simulink model "my_safety"  (R2023b)
settings: Solver=FixedStepAuto  StartTime=0.0  StopTime=inf  RelTol=1e-3
undefined symbols (not defined in the file): Alt, Button, Lat, Lon, recfin, Xa, Ya, Yg, Za
libraries: simulink x12, androiduilib x8, androidsensorlib x3, androidaudiovideolib x2, androidcommunicationlib x1
settings Model: Creator=salon  LastModifiedBy=salon
settings OptimizationCC: EnhancedBackFolding=on  PassReuseOutputArgsAs=Individual arguments  ZeroExternalMemoryAtStartup=off  ZeroInternalMemoryAtStartup=off  MaxStackSize=64  OptimizeBlockOrder=speed  DifferentSizesBufferReuse=on  OptimizationCustomize=off  EfficientTunableParamExpr=on
settings DebuggingCC: ParameterTunabilityLossMsg=error
settings HardwareCC: ProdBitPerPointer=32  ProdBitPerSizeT=32  ProdBitPerPtrDiffT=32  ProdLargestAtomicInteger=Long  ProdLargestAtomicFloat=Double  ProdWordSize=32  ProdHWDeviceType=ARM Compatible->ARM Cortex  UseEmbeddedCoderFeatures=off  UseSimulinkCoderFeatures=off
settings SFSimCC: MATLABDynamicMemAlloc=off
settings RTWCC: Description=Embedded Coder  SystemTargetFile=ert.tlc  HardwareBoard=Android Device  TLCOptions="-aInlineSetEventsForThisBaseRateFcn=TLC_FALSE -aSuppressMultiTaskScheduler=TLC_FALSE  -aRateBasedStepFcn=0"  TemplateMakefile=ert_default_tmf  RTWVerbose=off  Toolchain=Android SDK/NDK Tools
settings CodeAppCC: ForceParamTrailComments=on  IgnoreCustomStorageClasses=off  OperatorAnnotations=on  SimulinkDataObjDesc=on  SFDataObjDesc=on  InsertBlockDesc=on
settings ERTTargetCC: SupportNonInlinedSFcns=on

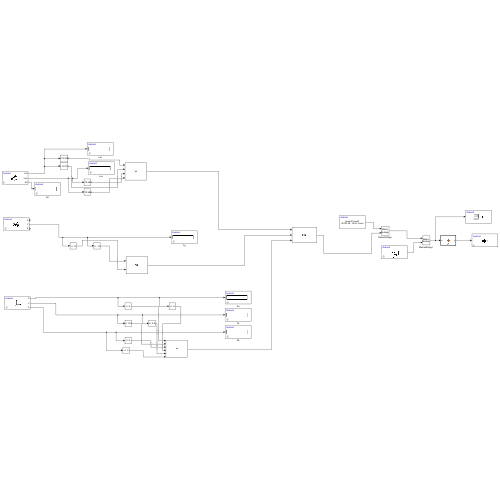
[thumbnail: Simulink's stored preview of the top-level diagram]
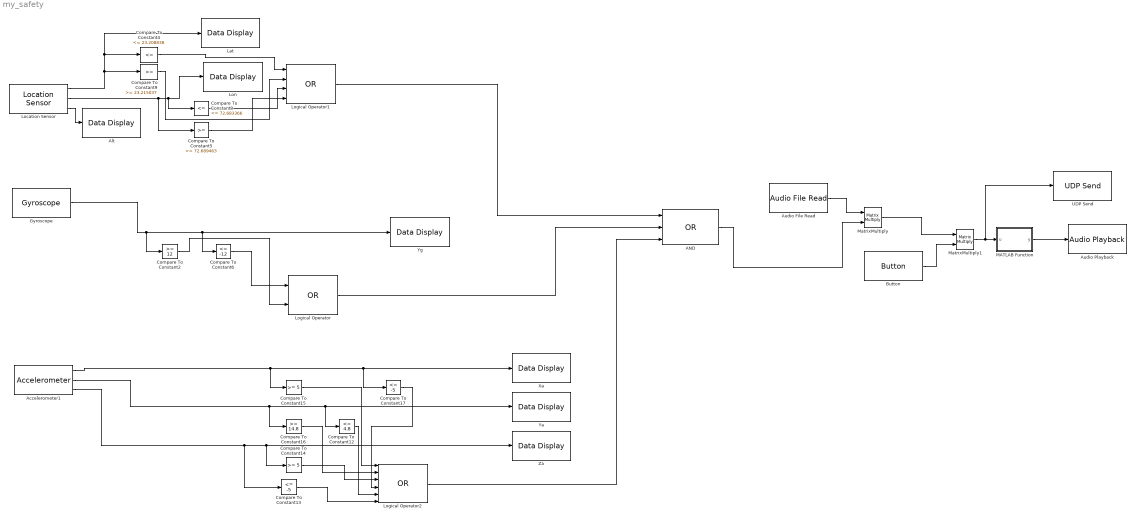
== system my_safety ==
  AND : Logic  Operator=OR  Inputs=3  AllPortsSameDT=off  OutDataTypeStr=boolean
  Accelerometer1 : androidsensorlib/Accelerometer  OutputVector=off  SampleTime=0.1  BlockPlatform=Android
  Alt : androiduilib/Data Display  DataDisplayId=recfin/Alt  Format=Float  Precision=6  SimulateUsing=Code generation  blockPlatform=Android
  Audio File Read : androidaudiovideolib/Audio File Read  FileName=C:\Users\salon\Downloads\beep-01a.mp3  FrameSize=4410
  Audio Playback : androidaudiovideolib/Audio Playback  SampleFreq=44100  AudioSamplingFreq=44100  SampleTime=0.1  DeviceStr=0  QueueDuration=0  BlockPlatform=Android
  Button : androiduilib/Button  ButtonState=Pressed  ButtonId=recfin/Button  State=on  SampleTime=0.1  BlockPlatform=Android
  Compare To Constant12 : simulink/Logic and Bit Operations/Compare To Constant  relop=<=  const=4.8  OutDataTypeStr=boolean
  Compare To Constant13 : simulink/Logic and Bit Operations/Compare To Constant  relop=<=  const=-5  OutDataTypeStr=boolean
  Compare To Constant14 : simulink/Logic and Bit Operations/Compare To Constant  relop=>=  const=5  OutDataTypeStr=boolean
  Compare To Constant15 : simulink/Logic and Bit Operations/Compare To Constant  relop=>=  const=5  OutDataTypeStr=boolean
  Compare To Constant16 : simulink/Logic and Bit Operations/Compare To Constant  relop=>=  const=14.8  OutDataTypeStr=boolean
  Compare To Constant17 : simulink/Logic and Bit Operations/Compare To Constant  relop=<=  const=-5  OutDataTypeStr=boolean
  Compare To Constant2 : simulink/Logic and Bit Operations/Compare To Constant  relop=>=  const=12  OutDataTypeStr=boolean
  Compare To Constant4 : simulink/Logic and Bit Operations/Compare To Constant  relop=<=  const=23.208838  OutDataTypeStr=boolean
  Compare To Constant5 : simulink/Logic and Bit Operations/Compare To Constant  relop=>=  const=72.689463  OutDataTypeStr=boolean
  Compare To Constant6 : simulink/Logic and Bit Operations/Compare To Constant  relop=<=  const=-12  OutDataTypeStr=boolean
  Compare To Constant8 : simulink/Logic and Bit Operations/Compare To Constant  relop=<=  const=72.683366  OutDataTypeStr=boolean
  Compare To Constant9 : simulink/Logic and Bit Operations/Compare To Constant  relop=>=  const=23.215037  OutDataTypeStr=boolean
  Gyroscope : androidsensorlib/Gyroscope  OutputVector=off  SampleTime=0.1  BlockPlatform=Android
  Lat : androiduilib/Data Display  DataDisplayId=recfin/Lat  Format=Float  Precision=6  SimulateUsing=Code generation  blockPlatform=Android
  Location Sensor : androidsensorlib/Location Sensor  OutputVector=off  SampleTime=0.1  BlockPlatform=Android
  Logical Operator : Logic  Operator=OR  AllPortsSameDT=off  OutDataTypeStr=boolean
  Logical Operator1 : Logic  Operator=OR  Inputs=4  AllPortsSameDT=off  OutDataTypeStr=boolean
  Logical Operator2 : Logic  Operator=OR  Inputs=6  AllPortsSameDT=off  OutDataTypeStr=boolean
  Lon : androiduilib/Data Display  DataDisplayId=recfin/Lon  Format=Float  Precision=6  SimulateUsing=Code generation  blockPlatform=Android
  MATLAB Function : MATLAB Function  TreatAsAtomicUnit=on
  MatrixMultiply : Product  Multiplication=Matrix(*)
  MatrixMultiply1 : Product  Multiplication=Matrix(*)
  UDP Send : androidcommunicationlib/UDP Send  remoteURL='10.7.9.45'  remotePort=8000  localURL='0.0.0.0'  localPortSource=Automatically determine  localPort=-1  sampletime=-1  blockPlatform=Android  separateLengthPort=0
  Xa : androiduilib/Data Display  DataDisplayId=recfin/Xa  Format=Float  Precision=6  SimulateUsing=Code generation  blockPlatform=Android
  Ya : androiduilib/Data Display  DataDisplayId=recfin/Ya  Format=Float  Precision=6  SimulateUsing=Code generation  blockPlatform=Android
  Yg : androiduilib/Data Display  DataDisplayId=recfin/Yg  Format=Float  Precision=6  SimulateUsing=Code generation  blockPlatform=Android
  Za : androiduilib/Data Display  DataDisplayId=recfin/Za  Format=Float  Precision=6  SimulateUsing=Code generation  blockPlatform=Android
  wires:
  Gyroscope/2 -> Compare To Constant2/1, Compare To Constant6/1, Yg/1
  Location Sensor/2 -> Compare To Constant5/1, Compare To Constant8/1, Lon/1
  Location Sensor/3 -> Alt/1
  Compare To Constant2/1 -> Logical Operator/2
  Location Sensor/1 -> Compare To Constant9/1, Lat/1, Compare To Constant4/1
  Compare To Constant4/1 -> Logical Operator1/1
  Compare To Constant9/1 -> Logical Operator1/2
  Compare To Constant8/1 -> Logical Operator1/3
  Compare To Constant5/1 -> Logical Operator1/4
  Logical Operator1/1 -> AND/1
  Audio File Read/1 -> MatrixMultiply/1
  AND/1 -> MatrixMultiply/2
  MatrixMultiply/1 -> MatrixMultiply1/1
  Button/1 -> MatrixMultiply1/2
  Compare To Constant6/1 -> Logical Operator/1
  Compare To Constant13/1 -> Logical Operator2/6
  Compare To Constant16/1 -> Logical Operator2/2
  Compare To Constant15/1 -> Logical Operator2/1
  Accelerometer1/2 -> Compare To Constant16/1, Ya/1, Compare To Constant12/1
  Accelerometer1/1 -> Compare To Constant15/1, Xa/1, Compare To Constant17/1
  Compare To Constant12/1 -> Logical Operator2/5
  Accelerometer1/3 -> Compare To Constant13/1, Za/1, Compare To Constant14/1
  Compare To Constant17/1 -> Logical Operator2/4
  Compare To Constant14/1 -> Logical Operator2/3
  Logical Operator/1 -> AND/2
  Logical Operator2/1 -> AND/3
  MATLAB Function/1(y) -> Audio Playback/1
  MatrixMultiply1/1 -> MATLAB Function/1(u), UDP Send/1

== matlab function my_safety/MATLAB Function ==
  data: u input; y output
function y = fcn(u)
    if isequal(size(u), [4410, 1])
        y = [u, u];
    else
        error('Input size must be 4410x1.');
    end
end
